simulink model "lab_3_task_2_simulink"  (R2025b)
settings: Solver=ode5  StartTime=0.0  StopTime=t_end  FixedStep=0.1  RelTol=1e-3
values from neighbouring files (symbols this model uses):
  I = diag([ix iy iz])    [lab_3_task_3.m]    (also in lab_4_task_3.m; lab_5_task_1.m; lab_5_task_2.m; lab_6_task_1.m = diag([ ix iy iz ]))
  w = simout.w.Data    [lab_3_task_3.m]    (also in lab_4_task_3.m; lab_5_task_1.m; lab_5_task_2.m; lab_6_task_1.m)
libraries: matrix_library x1
settings Model: Creator=User  LastModifiedBy=User

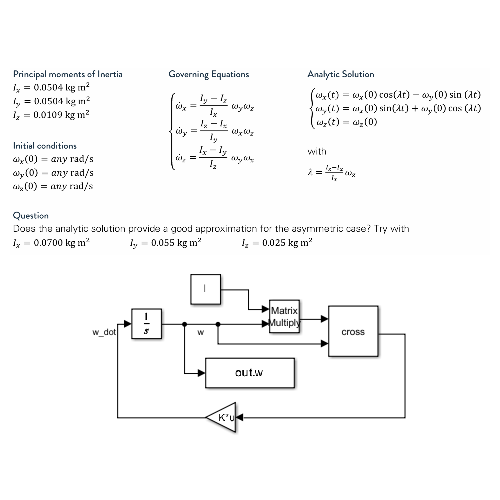
[thumbnail: Simulink's stored preview of the top-level diagram]
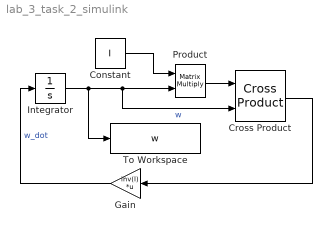
== system lab_3_task_2_simulink ==
  Constant : Constant  Value=I
  Cross Product : matrix_library/Cross Product
  Gain : Gain  Gain=inv(I)  Multiplication=Matrix(K*u)
  Integrator : Integrator  InitialCondition=w
  Product : Product  Multiplication=Matrix(*)
  To Workspace : ToWorkspace  VariableName=w  SaveFormat=Timeseries  SampleTime=-1
  wires:
  Integrator/1 -> To Workspace/1, Cross Product/2, Product/2  "w"
  Cross Product/1 -> Gain/1
  Constant/1 -> Product/1
  Product/1 -> Cross Product/1
  Gain/1 -> Integrator/1  "w_dot"
